simulink model "quadrotor_strategy_rl_v2"  (R2026a)
settings: Solver=ode4  StopTime=quad_stop_time  FixedStep=0.02
undefined symbols (not defined in the file): quad_model_id, quad_param_vec, quad_scenario_id, quad_x0
Description:
  | RL-v2策略模型：固定使用前瞻残差强化学习补偿策略。
settings Model: Creator=audib  LastModifiedBy=audib

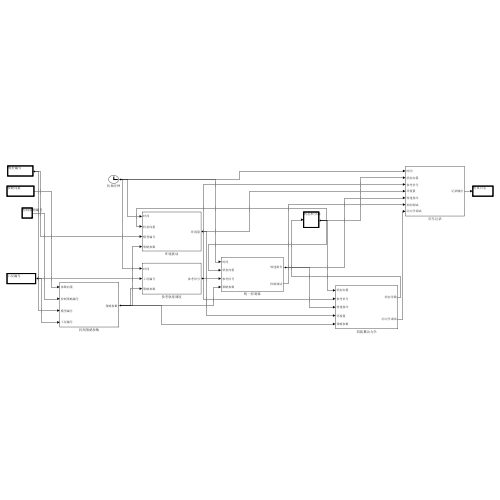
[thumbnail: Simulink's stored preview of the top-level diagram]
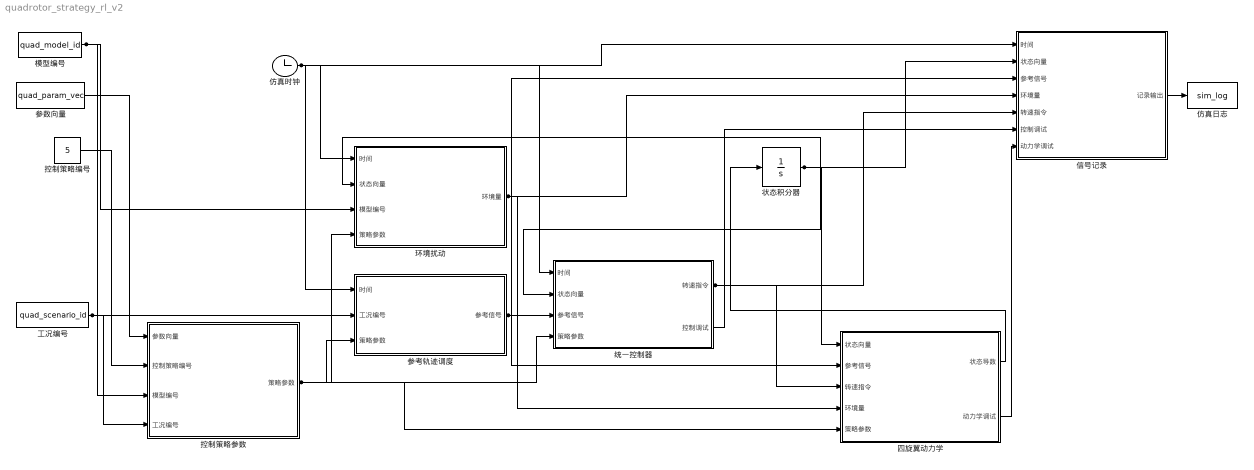
== system quadrotor_strategy_rl_v2 ==
  仿真日志 : ToWorkspace  VariableName=sim_log  SampleTime=-1
  仿真时钟 : Clock
  信号记录 : Subsystem
  参数向量 : Constant  Value=quad_param_vec
  参考轨迹调度 : Subsystem
  四旋翼动力学 : Subsystem
  工况编号 : Constant  Value=quad_scenario_id
  控制策略参数 : Subsystem
  控制策略编号 : Constant  Value=5
  模型编号 : Constant  Value=quad_model_id
  状态积分器 : Integrator  InitialCondition=quad_x0
  环境扰动 : Subsystem
  统一控制器 : Subsystem
  wires:
  控制策略参数/1(策略参数) -> 四旋翼动力学/5(策略参数), 统一控制器/4(策略参数), 环境扰动/4(策略参数), 参考轨迹调度/3(策略参数)
  模型编号/1 -> 环境扰动/3(模型编号), 控制策略参数/3(模型编号)
  控制策略编号/1 -> 控制策略参数/2(控制策略编号)
  工况编号/1 -> 参考轨迹调度/2(工况编号), 控制策略参数/4(工况编号)
  参数向量/1 -> 控制策略参数/1(参数向量)
  仿真时钟/1 -> 信号记录/1(时间), 环境扰动/1(时间), 参考轨迹调度/1(时间), 统一控制器/1(时间)
  环境扰动/1(环境量) -> 四旋翼动力学/4(环境量), 信号记录/4(环境量)
  参考轨迹调度/1(参考信号) -> 四旋翼动力学/2(参考信号), 统一控制器/3(参考信号), 信号记录/3(参考信号)
  统一控制器/1(转速指令) -> 四旋翼动力学/3(转速指令), 信号记录/5(转速指令)
  统一控制器/2(控制调试) -> 信号记录/6(控制调试)
  状态积分器/1 -> 环境扰动/2(状态向量), 统一控制器/2(状态向量), 信号记录/2(状态向量), 四旋翼动力学/1(状态向量)
  四旋翼动力学/1(状态导数) -> 状态积分器/1
  四旋翼动力学/2(动力学调试) -> 信号记录/7(动力学调试)
  信号记录/1(记录输出) -> 仿真日志/1

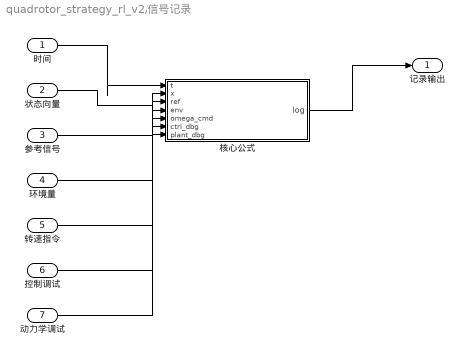
== system quadrotor_strategy_rl_v2/信号记录 ==
  时间 : Inport
  状态向量 : Inport  Port=2
  参考信号 : Inport  Port=3
  环境量 : Inport  Port=4
  转速指令 : Inport  Port=5
  控制调试 : Inport  Port=6
  动力学调试 : Inport  Port=7
  核心公式 : MATLAB Function  TreatAsAtomicUnit=on
  记录输出 : Outport
  wires:
  时间/1 -> 核心公式/1(t)
  状态向量/1 -> 核心公式/2(x)
  参考信号/1 -> 核心公式/3(ref)
  环境量/1 -> 核心公式/4(env)
  转速指令/1 -> 核心公式/5(omega_cmd)
  控制调试/1 -> 核心公式/6(ctrl_dbg)
  动力学调试/1 -> 核心公式/7(plant_dbg)
  核心公式/1(log) -> 记录输出/1

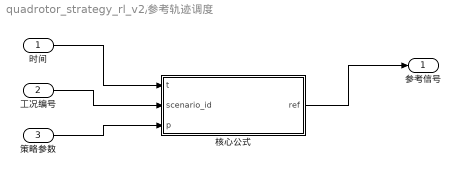
== system quadrotor_strategy_rl_v2/参考轨迹调度 ==
  时间 : Inport
  工况编号 : Inport  Port=2
  策略参数 : Inport  Port=3
  核心公式 : MATLAB Function  TreatAsAtomicUnit=on
  参考信号 : Outport
  wires:
  时间/1 -> 核心公式/1(t)
  工况编号/1 -> 核心公式/2(scenario_id)
  策略参数/1 -> 核心公式/3(p)
  核心公式/1(ref) -> 参考信号/1

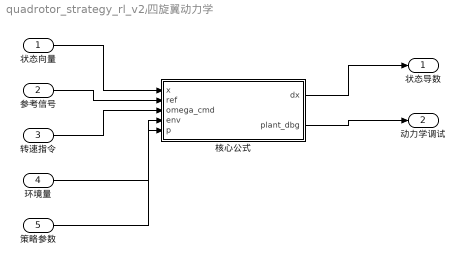
== system quadrotor_strategy_rl_v2/四旋翼动力学 ==
  状态向量 : Inport
  参考信号 : Inport  Port=2
  转速指令 : Inport  Port=3
  环境量 : Inport  Port=4
  策略参数 : Inport  Port=5
  核心公式 : MATLAB Function  TreatAsAtomicUnit=on
  状态导数 : Outport
  动力学调试 : Outport  Port=2
  wires:
  状态向量/1 -> 核心公式/1(x)
  参考信号/1 -> 核心公式/2(ref)
  转速指令/1 -> 核心公式/3(omega_cmd)
  环境量/1 -> 核心公式/4(env)
  策略参数/1 -> 核心公式/5(p)
  核心公式/1(dx) -> 状态导数/1
  核心公式/2(plant_dbg) -> 动力学调试/1

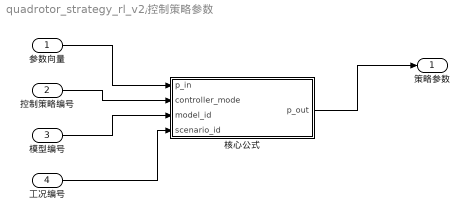
== system quadrotor_strategy_rl_v2/控制策略参数 ==
  参数向量 : Inport
  控制策略编号 : Inport  Port=2
  模型编号 : Inport  Port=3
  工况编号 : Inport  Port=4
  核心公式 : MATLAB Function  TreatAsAtomicUnit=on
  策略参数 : Outport
  wires:
  参数向量/1 -> 核心公式/1(p_in)
  控制策略编号/1 -> 核心公式/2(controller_mode)
  模型编号/1 -> 核心公式/3(model_id)
  工况编号/1 -> 核心公式/4(scenario_id)
  核心公式/1(p_out) -> 策略参数/1

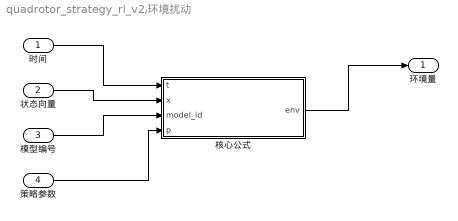
== system quadrotor_strategy_rl_v2/环境扰动 ==
  时间 : Inport
  状态向量 : Inport  Port=2
  模型编号 : Inport  Port=3
  策略参数 : Inport  Port=4
  核心公式 : MATLAB Function  TreatAsAtomicUnit=on
  环境量 : Outport
  wires:
  时间/1 -> 核心公式/1(t)
  状态向量/1 -> 核心公式/2(x)
  模型编号/1 -> 核心公式/3(model_id)
  策略参数/1 -> 核心公式/4(p)
  核心公式/1(env) -> 环境量/1

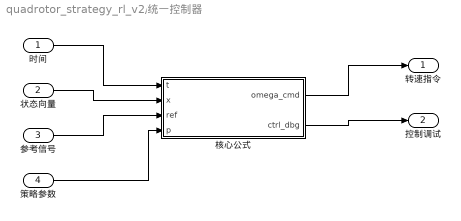
== system quadrotor_strategy_rl_v2/统一控制器 ==
  时间 : Inport
  状态向量 : Inport  Port=2
  参考信号 : Inport  Port=3
  策略参数 : Inport  Port=4
  核心公式 : MATLAB Function  TreatAsAtomicUnit=on
  转速指令 : Outport
  控制调试 : Outport  Port=2
  wires:
  时间/1 -> 核心公式/1(t)
  状态向量/1 -> 核心公式/2(x)
  参考信号/1 -> 核心公式/3(ref)
  策略参数/1 -> 核心公式/4(p)
  核心公式/1(omega_cmd) -> 转速指令/1
  核心公式/2(ctrl_dbg) -> 控制调试/1

== matlab function quadrotor_strategy_rl_v2/参考轨迹调度/核心公式 ==
  data: t input; ref output; scenario_id input; p input
function ref = fcn(t, scenario_id, p)
%#codegen
ref = quadrotor_reference_core(t, scenario_id, p);
end

== matlab function quadrotor_strategy_rl_v2/控制策略参数/核心公式 ==
  data: p_in input; p_out output; controller_mode input; model_id input; scenario_id input
function p_out = fcn(p_in, controller_mode, model_id, scenario_id)
%#codegen
p_out = p_in;
p_out(88) = scenario_id;
p_out(89) = controller_mode;
p_out(90) = model_id;
p_out(97) = 1.0;
p_out(121) = 2;
p_out(122) = 1;
p_out(123) = 0;
p_out(124) = -6.86119704952915;
p_out(125) = 0.0500108788797668;
p_out(126) = 0.0337752660167963;
p_out(127) = 0.753646783838056;
p_out(128) = -9.11635399313658;
p_out(129) = -11.2202478081658;
p_out(130) = 27.7126079862883;
p_out(131) = -3.39204159022625;
p_out(132) = -9.18194463550282;
p_out(133) = 20.853113158886;
p_out(134) = 5.58148365759711;
p_out(135) = -0.689052983590845;
p_out(136) = 7.30888787671349;
p_out(137) = -11.5541087341185;
p_out(138) = -2.87027800247676;
p_out(139) = -10.5908810760814;
p_out(140) = -10.9833843163086;
p_out(141) = 6.59414934249707;
p_out(142) = 0.887847169869395;
p_out(143) = -4.79342505777425;
p_out(144) = -0.660288335887544;
p_out(145) = -5.32901759298719;
p_out(146) = 3.68934199420782;
p_out(147) = 14.1963670384465;
p_out(148) = -12.9623750512863;
p_out(149) = 4.78667839707302;
p_out(150) = 8.03045709916537;
p_out(151) = -0.884076775746636;
p_out(152) = -5.76608582783721;
p_out(153) = 8.68603648386739;
p_out(154) = -19.0590323560531;
p_out(155) = 1.49334914126597;
p_out(156) = -3.40676328886257;
p_out(157) = 0.537495082889288;
p_out(158) = 0.257613835668793;
p_out(159) = -0.705692439511125;
p_out(160) = -1.49611680899209;
p_out(161) = -1.03167007904855;
p_out(162) = 3.45666455375646;
p_out(163) = -0.101129074268984;
p_out(164) = -0.903204441026648;
p_out(165) = 3.28806234732324;
p_out(166) = -0.1698513513579;
p_out(167) = -0.0438099196396888;
p_out(168) = 0.802645304982375;
p_out(169) = -1.35694627393171;
p_out(170) = -1.81802938474078;
p_out(171) = -1.20435359118041;
p_out(172) = 2.56024090984623;
p_out(173) = -0.154445864377946;
p_out(174) = -0.231183407110279;
p_out(175) = 0.13416260435219;
p_out(176) = 1.72263214958111;
p_out(177) = -0.0452464041549203;
p_out(178) = -1.65265125470729;
p_out(179) = 0.411778703707248;
p_out(180) = 0.0739603091775716;
p_out(181) = -1.3961344358248;
p_out(182) = 0.188476154143773;
p_out(183) = 0.0650470614725441;
p_out(184) = -0.0269230556456943;
p_out(185) = 0.236633018211585;
p_out(186) = 1.57744593284624;
p_out(187) = 0.386968095954971;
p_out(188) = 2.58693164639912;
p_out(189) = -0.157832405117312;
p_out(190) = -0.345710981909273;
p_out(191) = 0.228418588030457;
p_out(192) = 1.67349345027715;
p_out(193) = -0.0644828097642398;
p_out(194) = -1.6256464473036;
p_out(195) = 0.366802403364655;
p_out(196) = 0.0903919200991261;
p_out(197) = -1.42304912079196;
p_out(198) = 0.249073276274114;
p_out(199) = 0.0528326103157193;
p_out(200) = -0.0686074824350942;
p_out(201) = 0.268411157197038;
p_out(202) = 1.54610544040507;
p_out(203) = 0.399150742087529;
p_out(204) = -3.07576997327686;
p_out(205) = 3.83597223177954;
p_out(206) = -0.1370531285569;
p_out(207) = -0.100054023276282;
p_out(208) = -0.0865901426932431;
p_out(209) = 0.488367087019097;
p_out(210) = 0.544833774622096;
p_out(211) = 1.52224232548395;
p_out(212) = 0.23859101162589;
p_out(213) = 0.23859101162589;
p_out(214) = 0;
p_out(215) = 0.951614277797505;
p_out(216) = 0.991175204266177;
p_out(217) = 1.01077358358295;
p_out(218) = 1.01472572332057;
p_out(219) = 3;
p_out(220) = 0.0939738621053691;
p_out(221) = 0;
p_out(222) = 0;
p_out(223) = 0;
p_out(224) = 0;
p_out(225) = 0;
p_out(226) = 0;
p_out(227) = 0;
p_out(228) = 0;
p_out(229) = 0;
p_out(230) = 0;
p_out(231) = 0;
p_out(232) = 0;
p_out(233) = 0;
p_out(234) = 0;
p_out(235) = 0;
p_out(236) = 0;
p_out(237) = 0;
p_out(238) = 0;
p_out(239) = 0;
p_out(240) = 0;
end

== matlab function quadrotor_strategy_rl_v2/环境扰动/核心公式 ==
  data: t input; env output; x input; model_id input; p input
function env = fcn(t, x, model_id, p)
%#codegen
env = quadrotor_environment_core(t, x, model_id, p);
end

== matlab function quadrotor_strategy_rl_v2/统一控制器/核心公式 ==
  data: t input; omega_cmd output; x input; ref input; p input; ctrl_dbg output
function [omega_cmd, ctrl_dbg] = fcn(t, x, ref, p)
%#codegen
[omega_cmd, ctrl_dbg] = quadrotor_controller_core(t, x, ref, p);
end

== matlab function quadrotor_strategy_rl_v2/四旋翼动力学/核心公式 ==
  data: x input; dx output; ref input; omega_cmd input; env input; p input; plant_dbg output
function [dx, plant_dbg] = fcn(x, ref, omega_cmd, env, p)
%#codegen
[dx, plant_dbg] = quadrotor_rhs_core(x, ref, omega_cmd, env, p);
end

== matlab function quadrotor_strategy_rl_v2/信号记录/核心公式 ==
  data: t input; log output; x input; ref input; env input; omega_cmd input; ctrl_dbg input; plant_dbg input
function log = fcn(t, x, ref, env, omega_cmd, ctrl_dbg, plant_dbg)
%#codegen
log = quadrotor_pack_log_core(t, x, ref, env, omega_cmd, ctrl_dbg, plant_dbg);
end
